simulink model "ijc_template"  (R2020a)
settings: Solver=ode4  StartTime=0.0  StopTime=100  FixedStep=dt  RelTol=1e-3
settings Model: Creator=baradaran  LastModifiedBy=baradaran
settings DataIOCC: ReturnWorkspaceOutputs=off
settings DebuggingCC: ArithmeticOperatorsInVariantConditions=warning
settings SFSimCC: SimUseLocalCustomCode=off  CustomCodeUndefinedFunction=UseInterfaceOnly
settings RTWCC: RTWUseLocalCustomCode=off

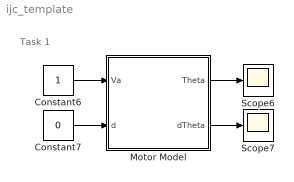
== system ijc_template ==
  note: Task 1
  Constant6 : Constant
  Constant7 : Constant  Value=0
  Motor Model : Subsystem
  Scope6 : Scope
  Scope7 : Scope
  wires:
  Constant6/1 -> Motor Model/1(Va)
  Constant7/1 -> Motor Model/2(d)
  Motor Model/1(Theta) -> Scope6/1
  Motor Model/2(dTheta) -> Scope7/1

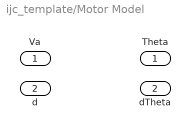
== system ijc_template/Motor Model ==
  Va : Inport
  d : Inport  Port=2
  Theta : Outport  VectorParamsAs1DForOutWhenUnconnected=off
  dTheta : Outport  Port=2  VectorParamsAs1DForOutWhenUnconnected=off
